simulink model "TST_TIntkVUs_DD"  (R2016b)
settings: Solver=FixedStepDiscrete  StartTime=0.0  StopTime=simTime  FixedStep=sampleTime  RelTol=1e-3
values from neighbouring files (symbols this model uses):
  testCase = 1    [initTST_TIntkVUs_DD_001.m]
libraries: UnitTest_Lib x5, simulink x2
settings Model: Creator=liangyunbo  LastModifiedBy=liangyunbo
settings DebuggingCC: SignalRangeChecking=error

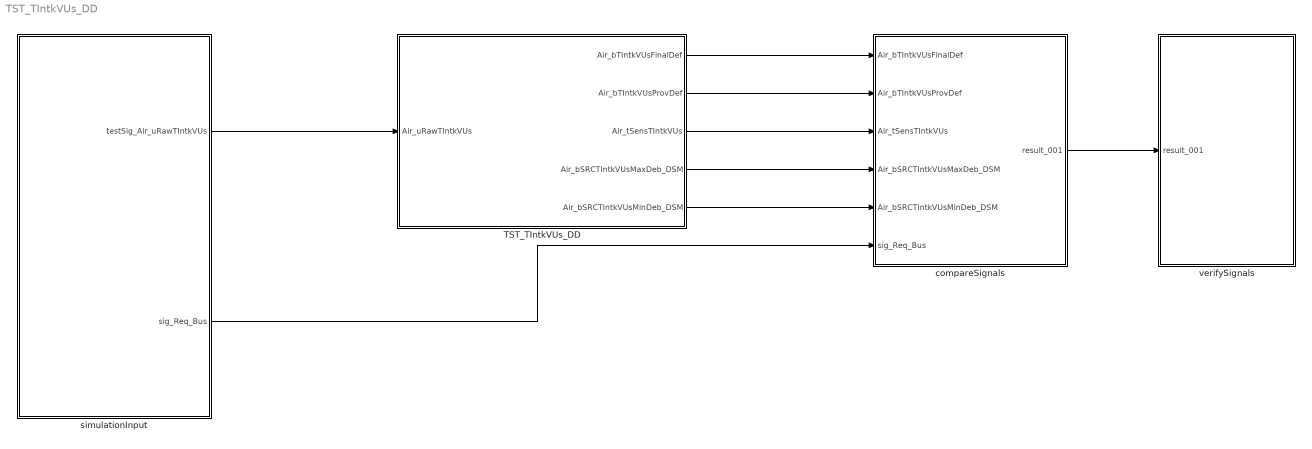
== system TST_TIntkVUs_DD ==
  TST_TIntkVUs_DD : Subsystem
  compareSignals : Subsystem
  simulationInput : Subsystem
  verifySignals : Subsystem
  wires:
  simulationInput/1(testSig_Air_uRawTIntkVUs) -> TST_TIntkVUs_DD/1(Air_uRawTIntkVUs)
  TST_TIntkVUs_DD/1(Air_bTIntkVUsFinalDef) -> compareSignals/1(Air_bTIntkVUsFinalDef)
  TST_TIntkVUs_DD/2(Air_bTIntkVUsProvDef) -> compareSignals/2(Air_bTIntkVUsProvDef)
  TST_TIntkVUs_DD/3(Air_tSensTIntkVUs) -> compareSignals/3(Air_tSensTIntkVUs)
  TST_TIntkVUs_DD/4(Air_bSRCTIntkVUsMaxDeb_DSM) -> compareSignals/4(Air_bSRCTIntkVUsMaxDeb_DSM)
  TST_TIntkVUs_DD/5(Air_bSRCTIntkVUsMinDeb_DSM) -> compareSignals/5(Air_bSRCTIntkVUsMinDeb_DSM)
  simulationInput/2(sig_Req_Bus) -> compareSignals/6(sig_Req_Bus)
  compareSignals/1(result_001) -> verifySignals/1(result_001)

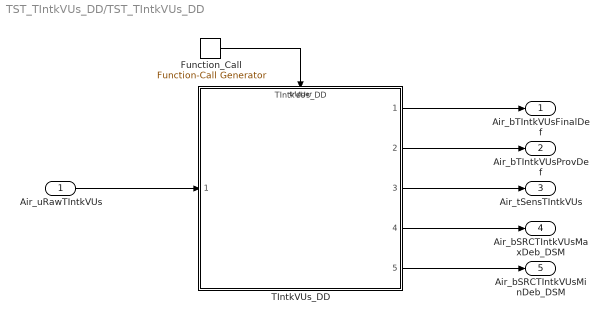
== system TST_TIntkVUs_DD/TST_TIntkVUs_DD ==
  Air_uRawTIntkVUs : Inport
  Function_Call : simulink/Ports & Subsystems/Function-Call Generator  sample_time=sampleTime  numberOfIterations=1
  TIntkVUs_DD : ModelReference  ModelNameDialog=TIntkVUs_DD  SimulationMode=Normal  ModelReferenceVersion=1.13  TriggerPortName=function  TriggerPortTriggerType=function-call  TriggerPortStatesWhenEnabling=held
  Air_bTIntkVUsFinalDef : Outport
  Air_bTIntkVUsProvDef : Outport  Port=2
  Air_tSensTIntkVUs : Outport  Port=3
  Air_bSRCTIntkVUsMaxDeb_DSM : Outport  Port=4
  Air_bSRCTIntkVUsMinDeb_DSM : Outport  Port=5
  wires:
  Function_Call/1 -> TIntkVUs_DD/Trigger
  Air_uRawTIntkVUs/1 -> TIntkVUs_DD/1
  TIntkVUs_DD/1 -> Air_bTIntkVUsFinalDef/1
  TIntkVUs_DD/2 -> Air_bTIntkVUsProvDef/1
  TIntkVUs_DD/3 -> Air_tSensTIntkVUs/1
  TIntkVUs_DD/4 -> Air_bSRCTIntkVUsMaxDeb_DSM/1
  TIntkVUs_DD/5 -> Air_bSRCTIntkVUsMinDeb_DSM/1

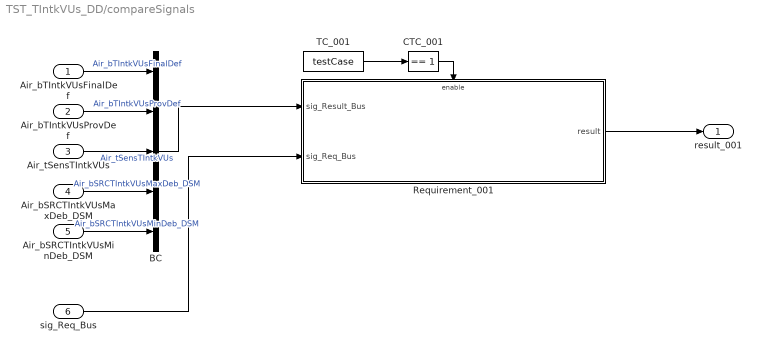
== system TST_TIntkVUs_DD/compareSignals ==
  Air_bTIntkVUsFinalDef : Inport
  Air_bTIntkVUsProvDef : Inport  Port=2
  Air_tSensTIntkVUs : Inport  Port=3
  Air_bSRCTIntkVUsMaxDeb_DSM : Inport  Port=4
  Air_bSRCTIntkVUsMinDeb_DSM : Inport  Port=5
  sig_Req_Bus : Inport  Port=6
  BC : BusCreator  Inputs=5
  CTC_001 : simulink/Logic and Bit Operations/Compare To Constant  relop===  const=1  OutDataTypeStr=boolean
  Requirement_001 : Subsystem
  TC_001 : Constant  Value=testCase
  result_001 : Outport
  wires:
  Air_bTIntkVUsFinalDef/1 -> BC/1  "Air_bTIntkVUsFinalDef"
  Air_bTIntkVUsProvDef/1 -> BC/2  "Air_bTIntkVUsProvDef"
  Air_tSensTIntkVUs/1 -> BC/3  "Air_tSensTIntkVUs"
  Air_bSRCTIntkVUsMaxDeb_DSM/1 -> BC/4  "Air_bSRCTIntkVUsMaxDeb_DSM"
  Air_bSRCTIntkVUsMinDeb_DSM/1 -> BC/5  "Air_bSRCTIntkVUsMinDeb_DSM"
  TC_001/1 -> CTC_001/1
  CTC_001/1 -> Requirement_001/Enable
  sig_Req_Bus/1 -> Requirement_001/2(sig_Req_Bus)
  BC/1 -> Requirement_001/1(sig_Result_Bus)
  Requirement_001/1(result) -> result_001/1

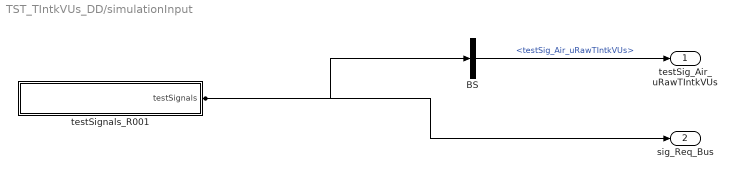
== system TST_TIntkVUs_DD/simulationInput ==
  BS : BusSelector  OutputSignals=testSig_Air_uRawTIntkVUs
  testSignals_R001 : Subsystem
  testSig_Air_uRawTIntkVUs : Outport
  sig_Req_Bus : Outport  Port=2
  wires:
  BS/1 -> testSig_Air_uRawTIntkVUs/1  "<testSig_Air_uRawTIntkVUs>"
  testSignals_R001/1(testSignals) -> BS/1, sig_Req_Bus/1

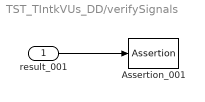
== system TST_TIntkVUs_DD/verifySignals ==
  result_001 : Inport
  Assertion_001 : Assertion  Enabled=off
  wires:
  result_001/1 -> Assertion_001/1

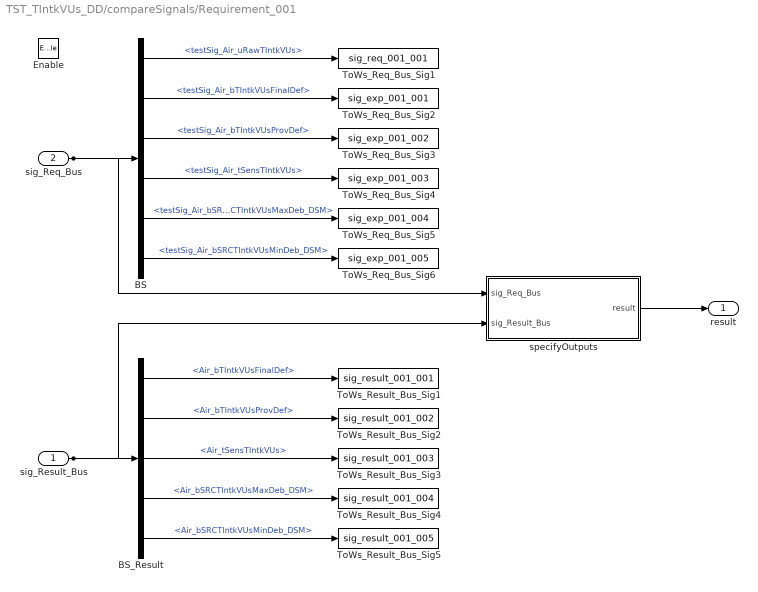
== system TST_TIntkVUs_DD/compareSignals/Requirement_001 ==
  sig_Result_Bus : Inport
  sig_Req_Bus : Inport  Port=2
  Enable : EnablePort
  BS : BusSelector  OutputSignals=testSig_Air_uRawTIntkVUs,testSig_Air_bTIntkVUsFinalDef,testSig_Air_bTIntkVUsProvDef,testSig_Air_tSensTIntkVUs,testSig_Air_bSRCTIntkVUsMaxDeb_DSM,testSig_Air_bSRCTIntkVUsMinDeb_DSM
  BS_Result : BusSelector  OutputSignals=Air_bTIntkVUsFinalDef,Air_bTIntkVUsProvDef,Air_tSensTIntkVUs,Air_bSRCTIntkVUsMaxDeb_DSM,Air_bSRCTIntkVUsMinDeb_DSM
  ToWs_Req_Bus_Sig1 : ToWorkspace  VariableName=sig_req_001_001  SaveFormat=Structure With Time
  ToWs_Req_Bus_Sig2 : ToWorkspace  VariableName=sig_exp_001_001  SaveFormat=Structure With Time
  ToWs_Req_Bus_Sig3 : ToWorkspace  VariableName=sig_exp_001_002  SaveFormat=Structure With Time
  ToWs_Req_Bus_Sig4 : ToWorkspace  VariableName=sig_exp_001_003  SaveFormat=Structure With Time
  ToWs_Req_Bus_Sig5 : ToWorkspace  VariableName=sig_exp_001_004  SaveFormat=Structure With Time
  ToWs_Req_Bus_Sig6 : ToWorkspace  VariableName=sig_exp_001_005  SaveFormat=Structure With Time
  ToWs_Result_Bus_Sig1 : ToWorkspace  VariableName=sig_result_001_001  SaveFormat=Structure With Time
  ToWs_Result_Bus_Sig2 : ToWorkspace  VariableName=sig_result_001_002  SaveFormat=Structure With Time
  ToWs_Result_Bus_Sig3 : ToWorkspace  VariableName=sig_result_001_003  SaveFormat=Structure With Time
  ToWs_Result_Bus_Sig4 : ToWorkspace  VariableName=sig_result_001_004  SaveFormat=Structure With Time
  ToWs_Result_Bus_Sig5 : ToWorkspace  VariableName=sig_result_001_005  SaveFormat=Structure With Time
  specifyOutputs : Subsystem
  result : Outport
  wires:
  sig_Req_Bus/1 -> BS/1, specifyOutputs/1(sig_Req_Bus)
  BS/1 -> ToWs_Req_Bus_Sig1/1  "<testSig_Air_uRawTIntkVUs>"
  BS/2 -> ToWs_Req_Bus_Sig2/1  "<testSig_Air_bTIntkVUsFinalDef>"
  BS/3 -> ToWs_Req_Bus_Sig3/1  "<testSig_Air_bTIntkVUsProvDef>"
  BS/4 -> ToWs_Req_Bus_Sig4/1  "<testSig_Air_tSensTIntkVUs>"
  BS/5 -> ToWs_Req_Bus_Sig5/1  "<testSig_Air_bSRCTIntkVUsMaxDeb_DSM>"
  BS/6 -> ToWs_Req_Bus_Sig6/1  "<testSig_Air_bSRCTIntkVUsMinDeb_DSM>"
  sig_Result_Bus/1 -> BS_Result/1, specifyOutputs/2(sig_Result_Bus)
  BS_Result/1 -> ToWs_Result_Bus_Sig1/1  "<Air_bTIntkVUsFinalDef>"
  BS_Result/2 -> ToWs_Result_Bus_Sig2/1  "<Air_bTIntkVUsProvDef>"
  BS_Result/3 -> ToWs_Result_Bus_Sig3/1  "<Air_tSensTIntkVUs>"
  BS_Result/4 -> ToWs_Result_Bus_Sig4/1  "<Air_bSRCTIntkVUsMaxDeb_DSM>"
  BS_Result/5 -> ToWs_Result_Bus_Sig5/1  "<Air_bSRCTIntkVUsMinDeb_DSM>"
  specifyOutputs/1(result) -> result/1

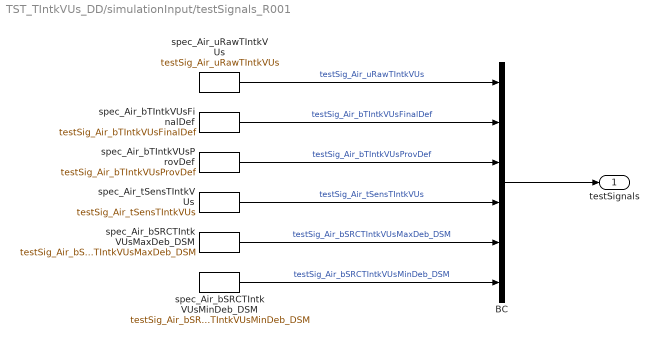
== system TST_TIntkVUs_DD/simulationInput/testSignals_R001 ==
  BC : BusCreator  Inputs=6
  spec_Air_bSRCTIntkVUsMaxDeb_DSM : FromWorkspace  VariableName=testSig_Air_bSRCTIntkVUsMaxDeb_DSM  Interpolate=off  OutputAfterFinalValue=Holding final value
  spec_Air_bSRCTIntkVUsMinDeb_DSM : FromWorkspace  VariableName=testSig_Air_bSRCTIntkVUsMinDeb_DSM  Interpolate=off  OutputAfterFinalValue=Holding final value
  spec_Air_bTIntkVUsFinalDef : FromWorkspace  VariableName=testSig_Air_bTIntkVUsFinalDef  Interpolate=off  OutputAfterFinalValue=Holding final value
  spec_Air_bTIntkVUsProvDef : FromWorkspace  VariableName=testSig_Air_bTIntkVUsProvDef  Interpolate=off  OutputAfterFinalValue=Holding final value
  spec_Air_tSensTIntkVUs : FromWorkspace  VariableName=testSig_Air_tSensTIntkVUs  Interpolate=off  OutputAfterFinalValue=Holding final value
  spec_Air_uRawTIntkVUs : FromWorkspace  VariableName=testSig_Air_uRawTIntkVUs  Interpolate=off  OutputAfterFinalValue=Holding final value
  testSignals : Outport
  wires:
  BC/1 -> testSignals/1
  spec_Air_uRawTIntkVUs/1 -> BC/1  "testSig_Air_uRawTIntkVUs"
  spec_Air_bTIntkVUsFinalDef/1 -> BC/2  "testSig_Air_bTIntkVUsFinalDef"
  spec_Air_bTIntkVUsProvDef/1 -> BC/3  "testSig_Air_bTIntkVUsProvDef"
  spec_Air_tSensTIntkVUs/1 -> BC/4  "testSig_Air_tSensTIntkVUs"
  spec_Air_bSRCTIntkVUsMaxDeb_DSM/1 -> BC/5  "testSig_Air_bSRCTIntkVUsMaxDeb_DSM"
  spec_Air_bSRCTIntkVUsMinDeb_DSM/1 -> BC/6  "testSig_Air_bSRCTIntkVUsMinDeb_DSM"

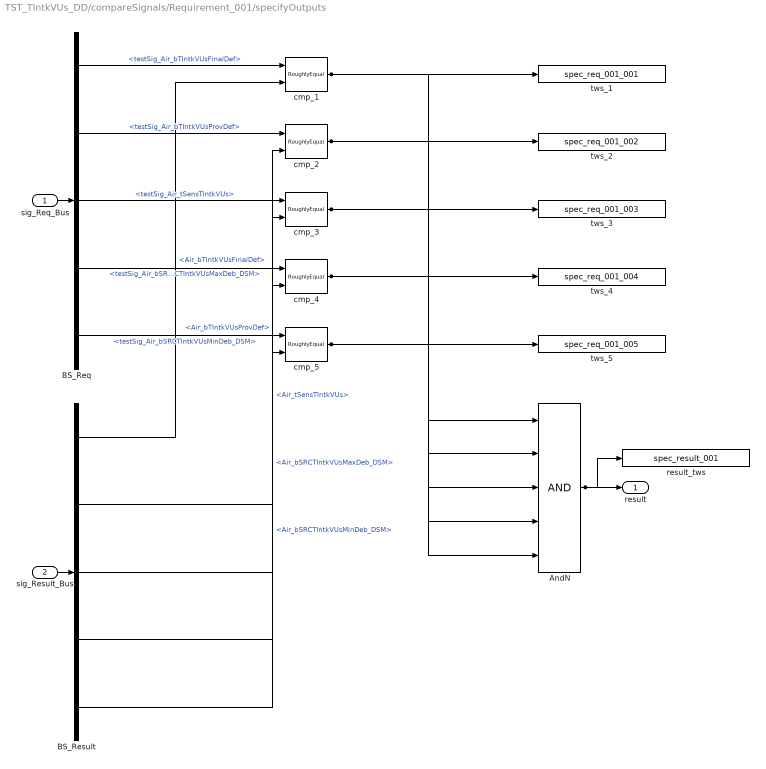
== system TST_TIntkVUs_DD/compareSignals/Requirement_001/specifyOutputs ==
  sig_Req_Bus : Inport
  sig_Result_Bus : Inport  Port=2
  AndN : Logic  Inputs=5
  BS_Req : BusSelector  OutputSignals=testSig_Air_bTIntkVUsFinalDef,testSig_Air_bTIntkVUsProvDef,testSig_Air_tSensTIntkVUs,testSig_Air_bSRCTIntkVUsMaxDeb_DSM,testSig_Air_bSRCTIntkVUsMinDeb_DSM
  BS_Result : BusSelector  OutputSignals=Air_bTIntkVUsFinalDef,Air_bTIntkVUsProvDef,Air_tSensTIntkVUs,Air_bSRCTIntkVUsMaxDeb_DSM,Air_bSRCTIntkVUsMinDeb_DSM
  cmp_{1..5} (5 alike) : UnitTest_Lib/RoughlyEqual  slope=0.1
  result_tws : ToWorkspace  VariableName=spec_result_001
  tws_1 : ToWorkspace  VariableName=spec_req_001_001
  tws_2 : ToWorkspace  VariableName=spec_req_001_002
  tws_3 : ToWorkspace  VariableName=spec_req_001_003
  tws_4 : ToWorkspace  VariableName=spec_req_001_004
  tws_5 : ToWorkspace  VariableName=spec_req_001_005
  result : Outport
  wires:
  sig_Req_Bus/1 -> BS_Req/1
  sig_Result_Bus/1 -> BS_Result/1
  AndN/1 -> result/1, result_tws/1
  BS_Req/1 -> cmp_1/1  "<testSig_Air_bTIntkVUsFinalDef>"
  BS_Result/1 -> cmp_1/2  "<Air_bTIntkVUsFinalDef>"
  cmp_1/1 -> tws_1/1, AndN/1
  BS_Req/2 -> cmp_2/1  "<testSig_Air_bTIntkVUsProvDef>"
  BS_Result/2 -> cmp_2/2  "<Air_bTIntkVUsProvDef>"
  cmp_2/1 -> tws_2/1, AndN/2
  BS_Req/3 -> cmp_3/1  "<testSig_Air_tSensTIntkVUs>"
  BS_Result/3 -> cmp_3/2  "<Air_tSensTIntkVUs>"
  cmp_3/1 -> tws_3/1, AndN/3
  BS_Req/4 -> cmp_4/1  "<testSig_Air_bSRCTIntkVUsMaxDeb_DSM>"
  BS_Result/4 -> cmp_4/2  "<Air_bSRCTIntkVUsMaxDeb_DSM>"
  cmp_4/1 -> tws_4/1, AndN/4
  BS_Req/5 -> cmp_5/1  "<testSig_Air_bSRCTIntkVUsMinDeb_DSM>"
  BS_Result/5 -> cmp_5/2  "<Air_bSRCTIntkVUsMinDeb_DSM>"
  cmp_5/1 -> tws_5/1, AndN/5
